simulink model "BehStorage"  (R2026a)
settings: Solver=VariableStepAuto
model workspace (MAT data in the model file):
  Capacity_bowls = 1000
  InitLevel_bowls = 500
settings Model: DataDictionary=BehParamsCommon.sldd  ParameterArgumentNames=Capacity_bowls,InitLevel_bowls  Creator=sarah  LastModifiedBy=sarah

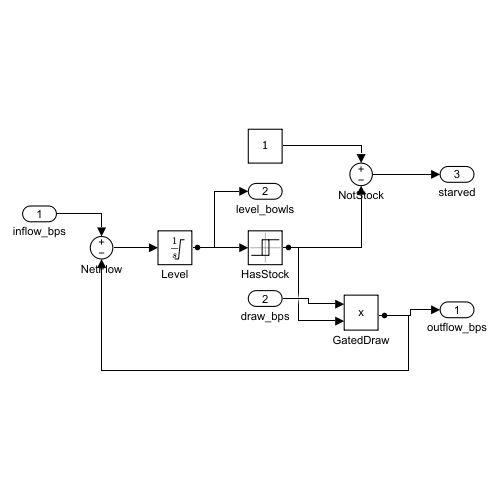
[thumbnail: Simulink's stored preview of the top-level diagram]
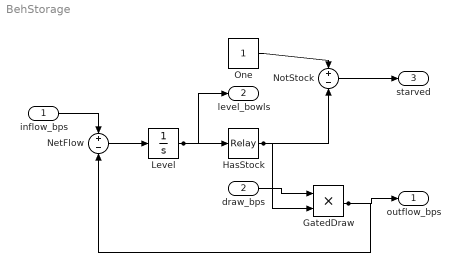
== system BehStorage ==
  inflow_bps : Inport
  draw_bps : Inport  Port=2
  GatedDraw : Product
  HasStock : Relay  OnSwitchValue=1.0  OffSwitchValue=0.1
  Level : Integrator  InitialCondition=InitLevel_bowls  LimitOutput=on  UpperSaturationLimit=Capacity_bowls  LowerSaturationLimit=0
  NetFlow : Sum  Inputs=+-
  NotStock : Sum  Inputs=+-
  One : Constant
  outflow_bps : Outport
  level_bowls : Outport  Port=2
  starved : Outport  Port=3
  wires:
  NotStock/1 -> starved/1
  One/1 -> NotStock/1
  HasStock/1 -> GatedDraw/2, NotStock/2
  draw_bps/1 -> GatedDraw/1
  Level/1 -> HasStock/1, level_bowls/1
  NetFlow/1 -> Level/1
  GatedDraw/1 -> NetFlow/2, outflow_bps/1
  inflow_bps/1 -> NetFlow/1
